simulink subsystem "ControlLedUnico"  (R2021b)
settings: Solver=VariableStepAuto  StartTime=0.0  StopTime=10.0  RelTol=1e-3
settings Model: Creator=yo  LastModifiedBy=yo

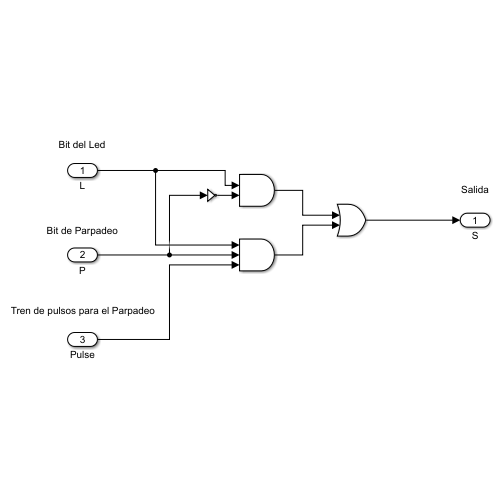
[thumbnail: Simulink's stored preview of the top-level diagram]
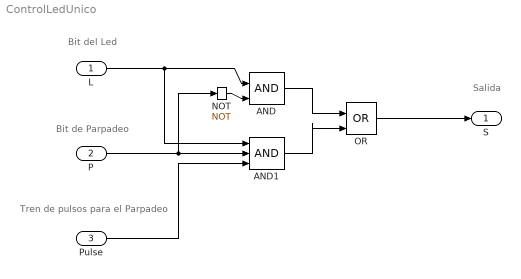
== system ControlLedUnico ==
  note: Bit del Led
  note: Bit de Parpadeo
  note: Tren de pulsos para el Parpadeo
  note: Salida
  L : Inport
  P : Inport  Port=2
  Pulse : Inport  Port=3
  AND : Logic  IconShape=distinctive  AllPortsSameDT=off  OutDataTypeStr=boolean
  AND1 : Logic  Inputs=3  IconShape=distinctive  AllPortsSameDT=off  OutDataTypeStr=boolean
  NOT : Logic  Operator=NOT  IconShape=distinctive  AllPortsSameDT=off  OutDataTypeStr=boolean
  OR : Logic  Operator=OR  IconShape=distinctive  AllPortsSameDT=off  OutDataTypeStr=boolean
  S : Outport
  wires:
  AND/1 -> OR/1
  Pulse/1 -> AND1/3
  P/1 -> AND1/2, NOT/1
  NOT/1 -> AND/2
  L/1 -> AND1/1, AND/1
  OR/1 -> S/1
  AND1/1 -> OR/2
